simulink model "SLModel"  (R2020a)
settings: Solver=VariableStepAuto  StartTime=0.0  StopTime=10.0  RelTol=1e-3
values from neighbouring files (symbols this model uses):
  c_ldeltar = 0.102    [Body.m]
  c_ndeltar = -0.065    [Body.m]
  h_init = longitudinal_data{1}.alt    [Body.m]
  lateral_data = datcomimport('lateral.out')    [Body.m]
  longitudinal_data = datcomimport('longitudinal.out')    [Body.m]
  mass = 4157    [Body.m]
  T_max = 22e3    (= 22000)    [Body.m]
  V_init = 328.6 * longitudinal_data{1}.mach    [Body.m]
libraries: aerolibasang x9, simulink_extras x8, aerolibadyn x4, shared6dof x1, aerolibatmos2 x1, aerolibtransform2 x1, aerolibconvert2 x1
settings Model: Creator=minec  LastModifiedBy=minec
settings DebuggingCC: AlgebraicLoopMsg=none

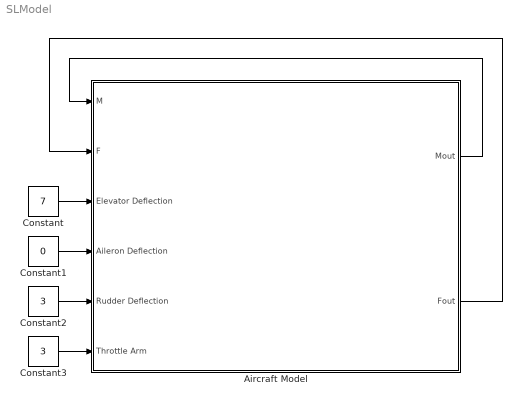
== system SLModel ==
  Aircraft Model : Subsystem
  Constant : Constant  Value=7
  Constant1 : Constant  Value=0
  Constant2 : Constant  Value=3
  Constant3 : Constant  Value=3
  wires:
  Constant1/1 -> Aircraft Model/4(Aileron Deflection)
  Constant/1 -> Aircraft Model/3(Elevator Deflection)
  Aircraft Model/1(Mout) -> Aircraft Model/1(M)
  Aircraft Model/2(Fout) -> Aircraft Model/2(F)
  Constant2/1 -> Aircraft Model/5(Rudder Deflection)
  Constant3/1 -> Aircraft Model/6(Throttle Arm)

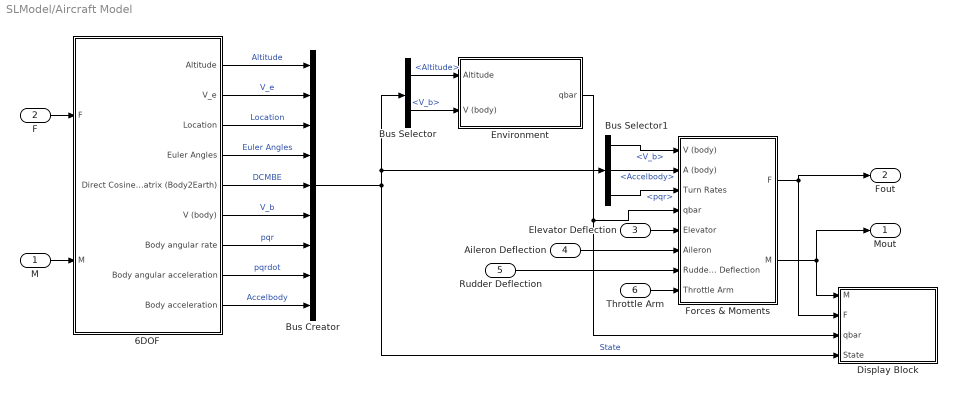
== system SLModel/Aircraft Model ==
  M : Inport
  F : Inport  Port=2
  Elevator Deflection : Inport  Port=3
  Aileron Deflection : Inport  Port=4
  Rudder Deflection : Inport  Port=5
  Throttle Arm : Inport  Port=6
  6DOF : Subsystem
  Bus Creator : BusCreator  Inputs=9
  Bus Selector : BusSelector  OutputSignals=Altitude,V_b
  Bus Selector1 : BusSelector  OutputSignals=V_b,Accelbody,pqr
  Display Block : Subsystem
  Environment : Subsystem
  Forces & Moments : Subsystem
  Mout : Outport
  Fout : Outport  Port=2
  wires:
  M/1 -> 6DOF/2(M)
  Forces & Moments/1(F) -> Fout/1, Display Block/2(F)
  Forces & Moments/2(M) -> Mout/1, Display Block/1(M)
  Environment/1(qbar) -> Display Block/3(qbar), Forces & Moments/4(qbar)
  F/1 -> 6DOF/1(F)
  Elevator Deflection/1 -> Forces & Moments/5(Elevator)
  Aileron Deflection/1 -> Forces & Moments/6(Aileron)
  6DOF/1(Altitude) -> Bus Creator/1  "Altitude"
  6DOF/2(V_e) -> Bus Creator/2  "V_e"
  6DOF/3(Location) -> Bus Creator/3  "Location"
  6DOF/4(Euler Angles) -> Bus Creator/4  "Euler Angles"
  6DOF/5(Direct Cosine Matrix (Body2Earth)) -> Bus Creator/5  "DCMBE"
  6DOF/6(V (body)) -> Bus Creator/6  "V_b"
  6DOF/7(Body angular rate) -> Bus Creator/7  "pqr"
  6DOF/8(Body angular acceleration) -> Bus Creator/8  "pqrdot"
  6DOF/9(Body acceleration) -> Bus Creator/9  "Accelbody"
  Bus Creator/1 -> Display Block/4(State), Bus Selector/1, Bus Selector1/1  "State"
  Bus Selector/1 -> Environment/1(Altitude)  "<Altitude>"
  Bus Selector/2 -> Environment/2(V (body))  "<V_b>"
  Bus Selector1/1 -> Forces & Moments/1(V (body))  "<V_b>"
  Bus Selector1/2 -> Forces & Moments/2(A (body))  "<Accelbody>"
  Bus Selector1/3 -> Forces & Moments/3(Turn Rates)  "<pqr>"
  Throttle Arm/1 -> Forces & Moments/8(Throttle Arm)
  Rudder Deflection/1 -> Forces & Moments/7(Rudder Deflection)

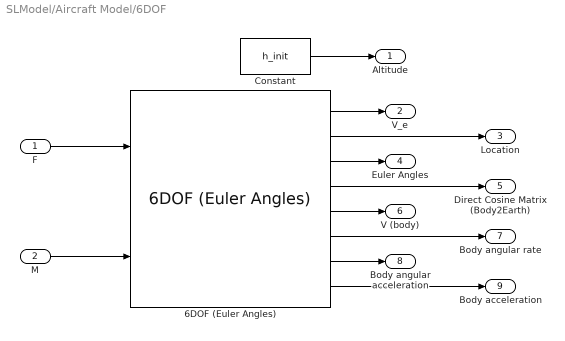
== system SLModel/Aircraft Model/6DOF ==
  F : Inport
  M : Inport  Port=2
  6DOF (Euler Angles) : shared6dof/6DOF (Euler Angles)  units=Metric (MKS)  mtype=Fixed  rep=Euler Angles  xme_0=[0 0 0]  Vm_0=[V_init 0 0]  eul_0=[0 0 0]  pm_0=[0 0 0]  mass_0=mass  mass_e=0.5  mass_f=2.0  inertia=Inertia  inertia_e=eye(3)  inertia_f=2*eye(3)  k_quat=1.0  vre_flag=on  abi_flag=off  aMode=0  xme_statename=''  Vm_statename=''  eul_statename=''  quat_statename=''  pm_statename=''  mass_statename=''
      settings: SourceProductBaseCode=AE,PW,MT,VE,VP
  Constant : Constant  Value=h_init
  Altitude : Outport
  V_e : Outport  Port=2
  Location : Outport  Port=3
  Euler Angles : Outport  Port=4
  Direct Cosine Matrix (Body2Earth) : Outport  Port=5
  V (body) : Outport  Port=6
  Body angular rate : Outport  Port=7
  Body angular acceleration : Outport  Port=8
  Body acceleration : Outport  Port=9
  wires:
  6DOF (Euler Angles)/5 -> V (body)/1
  Constant/1 -> Altitude/1
  F/1 -> 6DOF (Euler Angles)/1
  M/1 -> 6DOF (Euler Angles)/2
  6DOF (Euler Angles)/2 -> Location/1
  6DOF (Euler Angles)/3 -> Euler Angles/1
  6DOF (Euler Angles)/4 -> Direct Cosine Matrix (Body2Earth)/1
  6DOF (Euler Angles)/6 -> Body angular rate/1
  6DOF (Euler Angles)/7 -> Body angular acceleration/1
  6DOF (Euler Angles)/1 -> V_e/1
  6DOF (Euler Angles)/8 -> Body acceleration/1

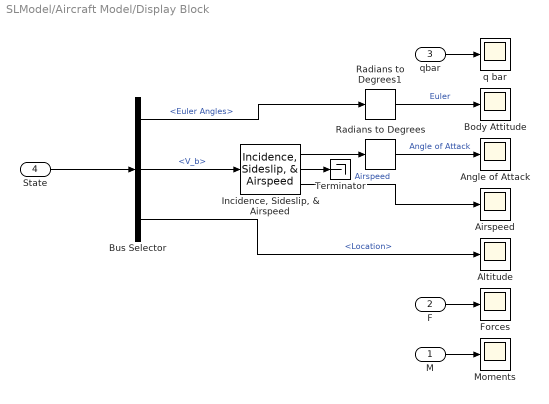
== system SLModel/Aircraft Model/Display Block ==
  M : Inport
  F : Inport  Port=2
  qbar : Inport  Port=3
  State : Inport  Port=4
  Airspeed : Scope
  Altitude : Scope
  Angle of Attack : Scope
  Body Attitude : Scope
  Bus Selector : BusSelector  OutputSignals=Euler Angles,V_b,Location
  Forces : Scope
  "Incidence, Sideslip, & Airspeed" : aerolibasang/Incidence, Sideslip, & Airspeed
  Moments : Scope
  Radians to Degrees : simulink_extras/Transformations/Radians to Degrees
  Radians to Degrees1 : simulink_extras/Transformations/Radians to Degrees
  Terminator : Terminator
  q bar : Scope
  wires:
  State/1 -> Bus Selector/1
  Bus Selector/2 -> "Incidence, Sideslip, & Airspeed"/1  "<V_b>"
  "Incidence, Sideslip, & Airspeed"/3 -> Airspeed/1  "Airspeed"
  "Incidence, Sideslip, & Airspeed"/2 -> Terminator/1
  F/1 -> Forces/1
  M/1 -> Moments/1
  Bus Selector/3 -> Altitude/1  "<Location>"
  "Incidence, Sideslip, & Airspeed"/1 -> Radians to Degrees/1
  Radians to Degrees/1 -> Angle of Attack/1  "Angle of Attack"
  Bus Selector/1 -> Radians to Degrees1/1  "<Euler Angles>"
  qbar/1 -> q bar/1
  Radians to Degrees1/1 -> Body Attitude/1  "Euler"

== system SLModel/Aircraft Model/Environment ==
  Altitude : Inport
  V (body) : Inport  Port=2
  Dynamic Pressure : aerolibasang/Dynamic Pressure
  ISA Atmosphere Model : aerolibatmos2/ISA Atmosphere Model  custom=off  g=9.80665  gamma=1.4  R=287.0531  L=0.0065  h_trop=11000  h_strat=20000  rho0=1.225  P0=101325  T0=288.15  h0=0
  Terminator : Terminator
  Terminator1 : Terminator
  Terminator2 : Terminator
  qbar : Outport
  wires:
  ISA Atmosphere Model/1 -> Terminator/1
  ISA Atmosphere Model/3 -> Terminator1/1
  ISA Atmosphere Model/2 -> Terminator2/1
  ISA Atmosphere Model/4 -> Dynamic Pressure/2
  V (body)/1 -> Dynamic Pressure/1
  Dynamic Pressure/1 -> qbar/1
  Altitude/1 -> ISA Atmosphere Model/1

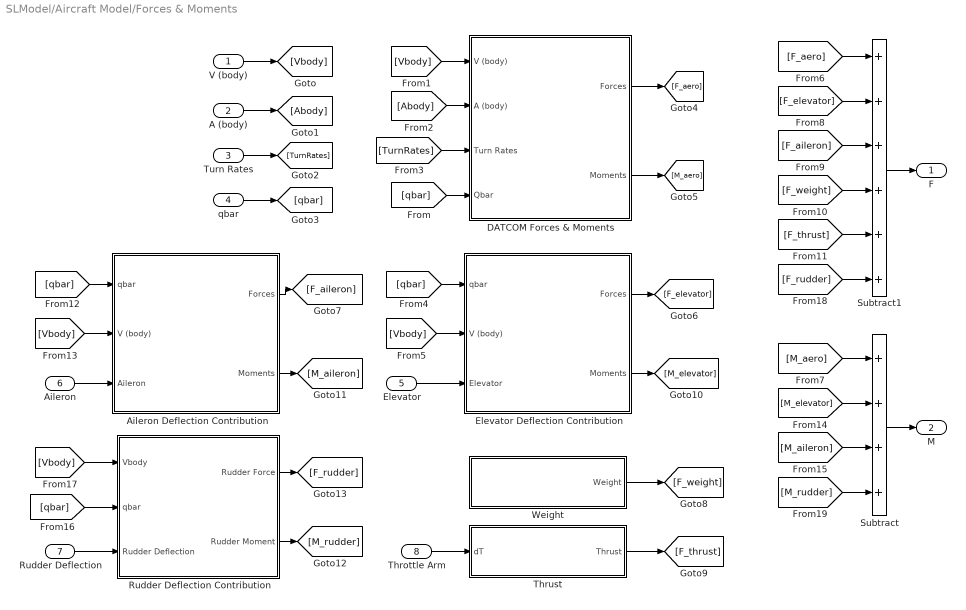
== system SLModel/Aircraft Model/Forces & Moments ==
  V (body) : Inport
  A (body) : Inport  Port=2
  Turn Rates : Inport  Port=3
  qbar : Inport  Port=4
  Elevator : Inport  Port=5
  Aileron : Inport  Port=6
  Rudder Deflection : Inport  Port=7
  Throttle Arm : Inport  Port=8
  Aileron Deflection Contribution : Subsystem
  DATCOM Forces & Moments : Subsystem
  Elevator Deflection Contribution : Subsystem
  Rudder Deflection Contribution : Subsystem
  Subtract : Sum  Inputs=++++
  Subtract1 : Sum  Inputs=++++++
  Thrust : Subsystem
  Weight : Subsystem
  F : Outport
  M : Outport  Port=2
  wires:
  [qbar] -> DATCOM Forces & Moments/4(Qbar)
  V (body)/1 -> [Vbody]
  Turn Rates/1 -> [TurnRates]
  A (body)/1 -> [Abody]
  qbar/1 -> [qbar]
  [Vbody] -> DATCOM Forces & Moments/1(V (body))
  [Abody] -> DATCOM Forces & Moments/2(A (body))
  [qbar] -> Elevator Deflection Contribution/1(qbar)
  [Vbody] -> Elevator Deflection Contribution/2(V (body))
  Elevator/1 -> Elevator Deflection Contribution/3(Elevator)
  [TurnRates] -> DATCOM Forces & Moments/3(Turn Rates)
  DATCOM Forces & Moments/1(Forces) -> [F_aero]
  DATCOM Forces & Moments/2(Moments) -> [M_aero]
  Elevator Deflection Contribution/1(Forces) -> [F_elevator]
  Aileron Deflection Contribution/1(Forces) -> [F_aileron]
  Weight/1(Weight) -> [F_weight]
  [Vbody] -> Aileron Deflection Contribution/2(V (body))
  [qbar] -> Aileron Deflection Contribution/1(qbar)
  Elevator Deflection Contribution/2(Moments) -> [M_elevator]
  Aileron Deflection Contribution/2(Moments) -> [M_aileron]
  [M_aero] -> Subtract/1
  [M_elevator] -> Subtract/2
  [M_aileron] -> Subtract/3
  Subtract/1 -> M/1
  [F_aero] -> Subtract1/1
  [F_elevator] -> Subtract1/2
  [F_aileron] -> Subtract1/3
  [F_weight] -> Subtract1/4
  [F_thrust] -> Subtract1/5
  Subtract1/1 -> F/1
  Aileron/1 -> Aileron Deflection Contribution/3(Aileron)
  Thrust/1(Thrust) -> [F_thrust]
  Throttle Arm/1 -> Thrust/1(dT)
  [qbar] -> Rudder Deflection Contribution/2(qbar)
  [Vbody] -> Rudder Deflection Contribution/1(Vbody)
  Rudder Deflection/1 -> Rudder Deflection Contribution/3(Rudder Deflection)
  Rudder Deflection Contribution/2(Rudder Moment) -> [M_rudder]
  Rudder Deflection Contribution/1(Rudder Force) -> [F_rudder]
  [M_rudder] -> Subtract/4
  [F_rudder] -> Subtract1/6

== system SLModel/Aircraft Model/Forces & Moments/Aileron Deflection Contribution ==
  qbar : Inport
  V (body) : Inport  Port=2
  Aileron : Inport  Port=3
  "Aerodynamic Forces and Moments " : aerolibadyn/Aerodynamic Forces and Moments   inputAxes=Body  outputForceAxes=Body  outputMomentAxes=Body  S=lateral_data{1}.sref  b=lateral_data{1}.blref  cbar=lateral_data{1}.cbar
  CP : Subsystem
  Coeffbody : Subsystem
  Constant : Constant  Value=[0 0 0]
  Forces : Outport
  Moments : Outport  Port=2
  wires:
  CP/1(CP) -> "Aerodynamic Forces and Moments "/4
  Aileron/1 -> Coeffbody/2(Aileron)
  Constant/1 -> "Aerodynamic Forces and Moments "/3
  Coeffbody/1(Coeff body) -> "Aerodynamic Forces and Moments "/1
  V (body)/1 -> Coeffbody/1(Vb), CP/1(V (body))
  "Aerodynamic Forces and Moments "/2 -> Moments/1
  "Aerodynamic Forces and Moments "/1 -> Forces/1
  qbar/1 -> "Aerodynamic Forces and Moments "/2

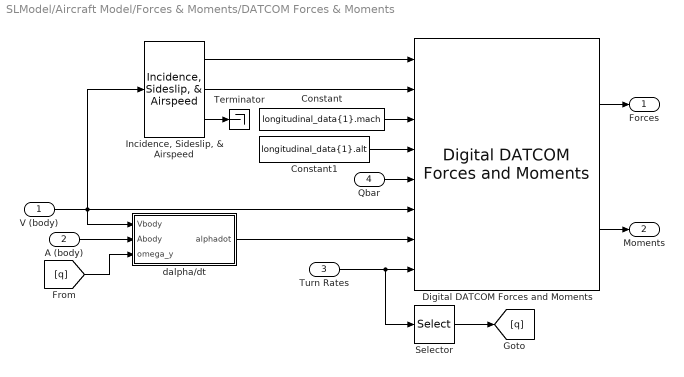
== system SLModel/Aircraft Model/Forces & Moments/DATCOM Forces & Moments ==
  V (body) : Inport
  A (body) : Inport  Port=2
  Turn Rates : Inport  Port=3
  Qbar : Inport  Port=4
  Constant : Constant  Value=longitudinal_data{1}.mach
  Constant1 : Constant  Value=longitudinal_data{1}.alt
  Digital DATCOM Forces and Moments : aerolibadyn/Digital DATCOM Forces and Moments  units=Metric (MKS)  dcase=longitudinal_data{1}  fmode=Body  buildno=0  imethod=Linear  emethod=Linear  rmethod=Linear Extrapolation  action=None
      settings: SourceProductBaseCode=AE
  "Incidence, Sideslip, & Airspeed" : aerolibasang/Incidence, Sideslip, & Airspeed
  Selector : Selector  InputPortWidth=3  IndexOptions=Index vector (dialog)  Indices=2  OutputSizes=1
  Terminator : Terminator
  dalpha/dt : Subsystem
  Forces : Outport
  Moments : Outport  Port=2
  wires:
  [q] -> dalpha/dt/3(omega_y)
  Selector/1 -> [q]
  Constant/1 -> Digital DATCOM Forces and Moments/3
  A (body)/1 -> dalpha/dt/2(Abody)
  "Incidence, Sideslip, & Airspeed"/2 -> Digital DATCOM Forces and Moments/2
  V (body)/1 -> "Incidence, Sideslip, & Airspeed"/1, Digital DATCOM Forces and Moments/6, dalpha/dt/1(Vbody)
  "Incidence, Sideslip, & Airspeed"/3 -> Terminator/1
  Digital DATCOM Forces and Moments/2 -> Moments/1
  Digital DATCOM Forces and Moments/1 -> Forces/1
  Qbar/1 -> Digital DATCOM Forces and Moments/5
  Turn Rates/1 -> Digital DATCOM Forces and Moments/8, Selector/1
  Constant1/1 -> Digital DATCOM Forces and Moments/4
  "Incidence, Sideslip, & Airspeed"/1 -> Digital DATCOM Forces and Moments/1
  dalpha/dt/1(alphadot) -> Digital DATCOM Forces and Moments/7

== system SLModel/Aircraft Model/Forces & Moments/Elevator Deflection Contribution ==
  qbar : Inport
  V (body) : Inport  Port=2
  Elevator : Inport  Port=3
  "Aerodynamic Forces and Moments " : aerolibadyn/Aerodynamic Forces and Moments   inputAxes=Body  outputForceAxes=Body  outputMomentAxes=Body  S=longitudinal_data{1}.sref  b=longitudinal_data{1}.blref  cbar=longitudinal_data{1}.cbar
  CP : Subsystem
  Coeffbody : Subsystem
  Constant : Constant  Value=[0 0 0]
  Forces : Outport
  Moments : Outport  Port=2
  wires:
  qbar/1 -> "Aerodynamic Forces and Moments "/2
  "Aerodynamic Forces and Moments "/1 -> Forces/1
  "Aerodynamic Forces and Moments "/2 -> Moments/1
  V (body)/1 -> CP/1(V (body)), Coeffbody/1(Vb)
  Coeffbody/1(Coeff body) -> "Aerodynamic Forces and Moments "/1
  Constant/1 -> "Aerodynamic Forces and Moments "/3
  Elevator/1 -> Coeffbody/2(Elevator)
  CP/1(CP) -> "Aerodynamic Forces and Moments "/4

== system SLModel/Aircraft Model/Forces & Moments/Rudder Deflection Contribution ==
  Vbody : Inport
  qbar : Inport  Port=2
  Rudder Deflection : Inport  Port=3
  Aerodynamic Forces and Moments 1 : aerolibadyn/Aerodynamic Forces and Moments   inputAxes=Body  outputForceAxes=Body  outputMomentAxes=Body  S=lateral_data{1}.sref  b=lateral_data{1}.blref  cbar=lateral_data{1}.cbar
  CP : Subsystem
  Coeffbody : Subsystem
  Constant : Constant  Value=[0 0 0]
  Rudder Force : Outport
  Rudder Moment : Outport  Port=2
  wires:
  qbar/1 -> Aerodynamic Forces and Moments 1/2
  Vbody/1 -> CP/1(V (body))
  Coeffbody/1(Coeff body) -> Aerodynamic Forces and Moments 1/1
  Constant/1 -> Aerodynamic Forces and Moments 1/3
  CP/1(CP) -> Aerodynamic Forces and Moments 1/4
  Aerodynamic Forces and Moments 1/1 -> Rudder Force/1
  Aerodynamic Forces and Moments 1/2 -> Rudder Moment/1
  Rudder Deflection/1 -> Coeffbody/1(Rudder)

== system SLModel/Aircraft Model/Forces & Moments/Thrust ==
  dT : Inport
  Constant : Constant  Value=T_max
  Ground : Ground
  Mux : Mux  Inputs=3
  Product : Product
  sigmoid : Subsystem
  Thrust : Outport
  wires:
  dT/1 -> sigmoid/1(dT)
  sigmoid/1(sigma(dT)) -> Product/1
  Constant/1 -> Product/2
  Product/1 -> Mux/1
  Ground/1 -> Mux/3, Mux/2
  Mux/1 -> Thrust/1

== system SLModel/Aircraft Model/Forces & Moments/Weight ==
  Constant : Constant  Value=mass
  Constant3 : Constant  Value=longitudinal_data{1}.alt
  Ground : Ground
  Length Conversion : aerolibconvert2/Length Conversion  IU=ft  OU=m
  Mux : Mux  Inputs=3
  Product : Product
  Selector1 : Selector  InputPortWidth=3  IndexOptions=Index vector (dialog)  Indices=3  OutputSizes=1
  Subsystem : Subsystem
  Weight : Outport
  wires:
  Constant3/1 -> Length Conversion/1
  Selector1/1 -> Product/1
  Length Conversion/1 -> Subsystem/1(Altitude)
  Subsystem/1(Gravitational Acceleration) -> Selector1/1
  Constant/1 -> Product/2
  Product/1 -> Mux/3
  Ground/1 -> Mux/2, Mux/1
  Mux/1 -> Weight/1

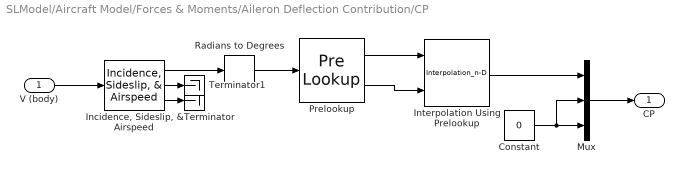
== system SLModel/Aircraft Model/Forces & Moments/Aileron Deflection Contribution/CP ==
  V (body) : Inport
  Constant : Constant  Value=0
  "Incidence, Sideslip, & Airspeed" : aerolibasang/Incidence, Sideslip, & Airspeed
  Interpolation Using Prelookup : Interpolation_n-D  NumberOfTableDimensions=1  Table=lateral_data{1}.xcp(~isnan(lateral_data{1}.xcp))*lateral_data{1}.cbar  InternalRulePriority=Speed
      settings: InputPortMap=u0,u1
  Mux : Mux  Inputs=3
  Prelookup : PreLookup  BreakpointsData=lateral_data{1}.alpha(~isnan(lateral_data{1}.xcp))  ExtrapMethod=Linear
  Radians to Degrees : simulink_extras/Transformations/Radians to Degrees
  Terminator : Terminator
  Terminator1 : Terminator
  CP : Outport
  wires:
  "Incidence, Sideslip, & Airspeed"/1 -> Radians to Degrees/1
  Radians to Degrees/1 -> Prelookup/1
  Mux/1 -> CP/1
  Constant/1 -> Mux/3, Mux/2
  Interpolation Using Prelookup/1 -> Mux/1
  Prelookup/2 -> Interpolation Using Prelookup/2
  Prelookup/1 -> Interpolation Using Prelookup/1
  "Incidence, Sideslip, & Airspeed"/2 -> Terminator1/1
  "Incidence, Sideslip, & Airspeed"/3 -> Terminator/1
  V (body)/1 -> "Incidence, Sideslip, & Airspeed"/1

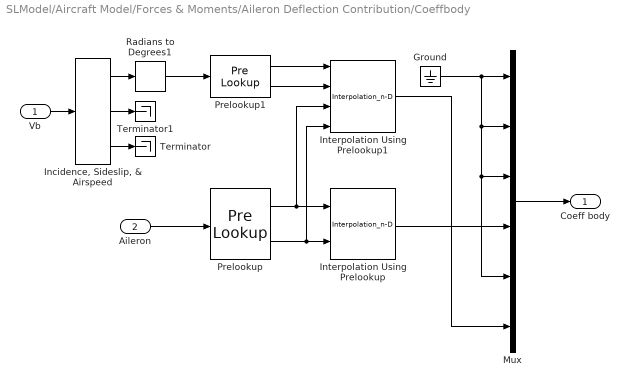
== system SLModel/Aircraft Model/Forces & Moments/Aileron Deflection Contribution/Coeffbody ==
  Vb : Inport
  Aileron : Inport  Port=2
  Ground : Ground
  "Incidence, Sideslip, & Airspeed" : aerolibasang/Incidence, Sideslip, & Airspeed
  Interpolation Using Prelookup : Interpolation_n-D  NumberOfTableDimensions=1  Table=lateral_data{1}.clroll  InternalRulePriority=Speed
      settings: InputPortMap=u0,u1
  Interpolation Using Prelookup1 : Interpolation_n-D  Table=lateral_data{1}.cn_asy  InternalRulePriority=Speed
  Mux : Mux  Inputs=6
  Prelookup : PreLookup  BreakpointsData=lateral_data{1}.deltal  ExtrapMethod=Linear
  Prelookup1 : PreLookup  BreakpointsData=lateral_data{1}.alpha  ExtrapMethod=Linear
  Radians to Degrees1 : simulink_extras/Transformations/Radians to Degrees
  Terminator : Terminator
  Terminator1 : Terminator
  Coeff body : Outport
  wires:
  Mux/1 -> Coeff body/1
  Vb/1 -> "Incidence, Sideslip, & Airspeed"/1
  Ground/1 -> Mux/5, Mux/3, Mux/2, Mux/1
  "Incidence, Sideslip, & Airspeed"/1 -> Radians to Degrees1/1
  "Incidence, Sideslip, & Airspeed"/3 -> Terminator/1
  Aileron/1 -> Prelookup/1
  Prelookup/1 -> Interpolation Using Prelookup1/3, Interpolation Using Prelookup/1
  Prelookup/2 -> Interpolation Using Prelookup1/4, Interpolation Using Prelookup/2
  Prelookup1/1 -> Interpolation Using Prelookup1/1
  Prelookup1/2 -> Interpolation Using Prelookup1/2
  Interpolation Using Prelookup/1 -> Mux/4
  Interpolation Using Prelookup1/1 -> Mux/6
  "Incidence, Sideslip, & Airspeed"/2 -> Terminator1/1
  Radians to Degrees1/1 -> Prelookup1/1

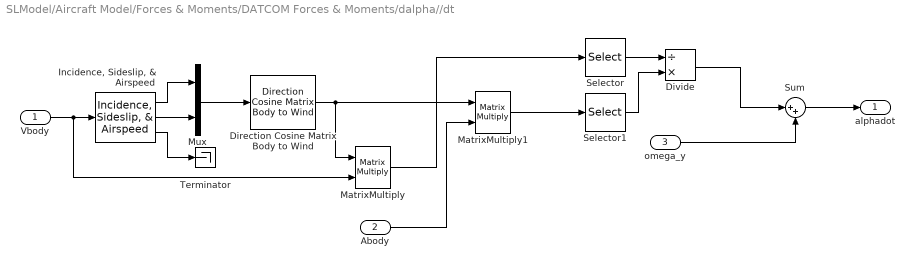
== system SLModel/Aircraft Model/Forces & Moments/DATCOM Forces & Moments/dalpha//dt ==
  Vbody : Inport
  Abody : Inport  Port=2
  omega_y : Inport  Port=3
  Direction Cosine Matrix Body to Wind : aerolibtransform2/Direction Cosine Matrix Body to Wind
      settings: SourceProductBaseCode=AE
  Divide : Product  Inputs=/*
  "Incidence, Sideslip, & Airspeed" : aerolibasang/Incidence, Sideslip, & Airspeed
  MatrixMultiply : Product  Multiplication=Matrix(*)
  MatrixMultiply1 : Product  Multiplication=Matrix(*)
  Mux : Mux  Inputs=2
  Selector : Selector  InputPortWidth=3  IndexOptions=Index vector (dialog)  Indices=1  OutputSizes=1
  Selector1 : Selector  InputPortWidth=3  IndexOptions=Index vector (dialog)  Indices=3  OutputSizes=1
  Sum : Sum  Inputs=|++
  Terminator : Terminator
  alphadot : Outport
  wires:
  Mux/1 -> Direction Cosine Matrix Body to Wind/1
  "Incidence, Sideslip, & Airspeed"/2 -> Mux/2
  "Incidence, Sideslip, & Airspeed"/1 -> Mux/1
  "Incidence, Sideslip, & Airspeed"/3 -> Terminator/1
  MatrixMultiply1/1 -> Selector1/1
  Abody/1 -> MatrixMultiply1/2
  MatrixMultiply/1 -> Selector/1
  Selector1/1 -> Divide/2
  Sum/1 -> alphadot/1
  Selector/1 -> Divide/1
  omega_y/1 -> Sum/2
  Direction Cosine Matrix Body to Wind/1 -> MatrixMultiply1/1, MatrixMultiply/1
  Vbody/1 -> MatrixMultiply/2, "Incidence, Sideslip, & Airspeed"/1
  Divide/1 -> Sum/1

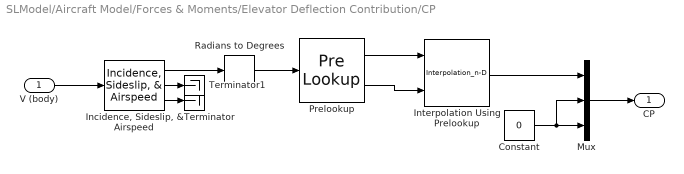
== system SLModel/Aircraft Model/Forces & Moments/Elevator Deflection Contribution/CP ==
  V (body) : Inport
  Constant : Constant  Value=0
  "Incidence, Sideslip, & Airspeed" : aerolibasang/Incidence, Sideslip, & Airspeed
  Interpolation Using Prelookup : Interpolation_n-D  NumberOfTableDimensions=1  Table=longitudinal_data{1}.xcp(~isnan(longitudinal_data{1}.xcp))*longitudinal_data{1}.cbar  InternalRulePriority=Speed
      settings: InputPortMap=u0,u1
  Mux : Mux  Inputs=3
  Prelookup : PreLookup  BreakpointsData=longitudinal_data{1}.alpha(~isnan(longitudinal_data{1}.xcp))  ExtrapMethod=Linear
  Radians to Degrees : simulink_extras/Transformations/Radians to Degrees
  Terminator : Terminator
  Terminator1 : Terminator
  CP : Outport
  wires:
  V (body)/1 -> "Incidence, Sideslip, & Airspeed"/1
  "Incidence, Sideslip, & Airspeed"/3 -> Terminator/1
  "Incidence, Sideslip, & Airspeed"/2 -> Terminator1/1
  Prelookup/1 -> Interpolation Using Prelookup/1
  Prelookup/2 -> Interpolation Using Prelookup/2
  Interpolation Using Prelookup/1 -> Mux/1
  Constant/1 -> Mux/2, Mux/3
  Mux/1 -> CP/1
  Radians to Degrees/1 -> Prelookup/1
  "Incidence, Sideslip, & Airspeed"/1 -> Radians to Degrees/1

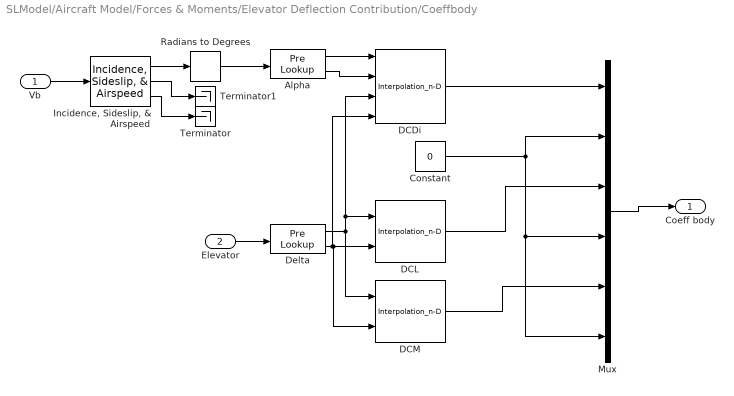
== system SLModel/Aircraft Model/Forces & Moments/Elevator Deflection Contribution/Coeffbody ==
  Vb : Inport
  Elevator : Inport  Port=2
  Alpha : PreLookup  BreakpointsData=longitudinal_data{1}.alpha  ExtrapMethod=Linear
  Constant : Constant  Value=0
  DCDi : Interpolation_n-D  Table=longitudinal_data{1}.dcdi_sym  InternalRulePriority=Speed
  DCL : Interpolation_n-D  NumberOfTableDimensions=1  Table=longitudinal_data{1}.dcl_sym  InternalRulePriority=Speed
      settings: InputPortMap=u0,u1
  DCM : Interpolation_n-D  NumberOfTableDimensions=1  Table=longitudinal_data{1}.dcm_sym  InternalRulePriority=Speed
      settings: InputPortMap=u0,u1
  Delta : PreLookup  BreakpointsData=longitudinal_data{1}.delta  ExtrapMethod=Linear
  "Incidence, Sideslip, & Airspeed" : aerolibasang/Incidence, Sideslip, & Airspeed
  Mux : Mux  Inputs=6
  Radians to Degrees : simulink_extras/Transformations/Radians to Degrees
  Terminator : Terminator
  Terminator1 : Terminator
  Coeff body : Outport
  wires:
  Vb/1 -> "Incidence, Sideslip, & Airspeed"/1
  "Incidence, Sideslip, & Airspeed"/2 -> Terminator1/1
  Mux/1 -> Coeff body/1
  "Incidence, Sideslip, & Airspeed"/3 -> Terminator/1
  Alpha/2 -> DCDi/2
  Alpha/1 -> DCDi/1
  Delta/2 -> DCM/2, DCL/2, DCDi/4
  Delta/1 -> DCDi/3, DCL/1, DCM/1
  DCDi/1 -> Mux/1
  Constant/1 -> Mux/6, Mux/4, Mux/2
  DCL/1 -> Mux/3
  DCM/1 -> Mux/5
  Radians to Degrees/1 -> Alpha/1
  "Incidence, Sideslip, & Airspeed"/1 -> Radians to Degrees/1
  Elevator/1 -> Delta/1

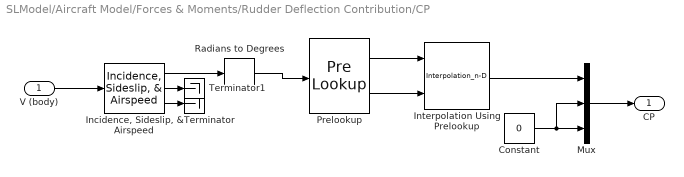
== system SLModel/Aircraft Model/Forces & Moments/Rudder Deflection Contribution/CP ==
  V (body) : Inport
  Constant : Constant  Value=0
  "Incidence, Sideslip, & Airspeed" : aerolibasang/Incidence, Sideslip, & Airspeed
  Interpolation Using Prelookup : Interpolation_n-D  NumberOfTableDimensions=1  Table=lateral_data{1}.xcp(~isnan(lateral_data{1}.xcp))*lateral_data{1}.cbar  InternalRulePriority=Speed
      settings: InputPortMap=u0,u1
  Mux : Mux  Inputs=3
  Prelookup : PreLookup  BreakpointsData=lateral_data{1}.alpha(~isnan(lateral_data{1}.xcp))  ExtrapMethod=Linear
  Radians to Degrees : simulink_extras/Transformations/Radians to Degrees
  Terminator : Terminator
  Terminator1 : Terminator
  CP : Outport
  wires:
  "Incidence, Sideslip, & Airspeed"/1 -> Radians to Degrees/1
  Radians to Degrees/1 -> Prelookup/1
  Mux/1 -> CP/1
  Constant/1 -> Mux/3, Mux/2
  Interpolation Using Prelookup/1 -> Mux/1
  Prelookup/2 -> Interpolation Using Prelookup/2
  Prelookup/1 -> Interpolation Using Prelookup/1
  "Incidence, Sideslip, & Airspeed"/2 -> Terminator1/1
  "Incidence, Sideslip, & Airspeed"/3 -> Terminator/1
  V (body)/1 -> "Incidence, Sideslip, & Airspeed"/1

== system SLModel/Aircraft Model/Forces & Moments/Rudder Deflection Contribution/Coeffbody ==
  Rudder : Inport
  Constant : Constant  Value=c_ndeltar
  Constant1 : Constant  Value=c_ldeltar
  Degrees to Radians : simulink_extras/Transformations/Degrees to Radians
  Ground : Ground
  Mux : Mux  Inputs=6
  Product : Product
  Product1 : Product
  Coeff body : Outport
  wires:
  Mux/1 -> Coeff body/1
  Ground/1 -> Mux/5, Mux/3, Mux/2, Mux/1
  Product/1 -> Mux/4
  Product1/1 -> Mux/6
  Constant1/1 -> Product/2
  Constant/1 -> Product1/2
  Degrees to Radians/1 -> Product1/1, Product/1
  Rudder/1 -> Degrees to Radians/1

== system SLModel/Aircraft Model/Forces & Moments/Thrust/sigmoid ==
  dT : Inport
  Constant : Constant
  Constant1 : Constant  Value=-2
  Constant2 : Constant
  Divide : Product  Inputs=*/
  Math Function : Math  SaturateOnIntegerOverflow=on
  Product : Product
  Sum : Sum  Inputs=+|+
  sigma(dT) : Outport
  wires:
  Constant/1 -> Divide/1
  Divide/1 -> sigma(dT)/1
  Constant1/1 -> Product/1
  dT/1 -> Product/2
  Product/1 -> Math Function/1
  Constant2/1 -> Sum/1
  Math Function/1 -> Sum/2
  Sum/1 -> Divide/2

== system SLModel/Aircraft Model/Forces & Moments/Weight/Subsystem ==
  Altitude : Inport
  Constant : Constant  Value=0
  Constant1 : Constant  Value=0
  Mux : Mux  Inputs=3
  "WGS84 Gravity Model  " : GravityWGS84
  Gravitational Acceleration : Outport
  wires:
  Altitude/1 -> Mux/3
  Mux/1 -> "WGS84 Gravity Model  "/1
  Constant/1 -> Mux/1
  Constant1/1 -> Mux/2
  "WGS84 Gravity Model  "/1 -> Gravitational Acceleration/1
